simulink model "simulator"  (R2021a)
settings: Solver=ode3  StartTime=0.0  StopTime=5000  FixedStep=1  RelTol=1e-3
InitFcn:
  | clear all
  | clc
  | 
  | %run config_Houston.m
  | run config_Malaga.m
  | 
  | load('PBNsim_buses');
StartFcn:
  | rng('shuffle');
undefined symbols (not defined in the file): entity, initX, instancedAC, m, n, WP, WPabort, WPnext, WPspeed
libraries: AC x23, aerolibactuator x3
(part 2 of 2)

== stateflow chart simulator/ATC/ATC ==
  state COMMUNICATIONS
    entry,during:
    msgProcess
    state msgProcess [function]
      (default) -> (junction 50)
      (junction 50) -> (junction 49) [order 1] : ACmsg
      (junction 48) -> (junction 50)
      (junction 50) -> (junction 53) [order 2]
      (junction 49) -> (junction 48) : {ACmsgProcess}
  data: ATCmsg output Bus: bus_ATMmsg; ACmsg input Bus: bus_ACmsg; WP parameter; WPspeed parameter; WPnext parameter; WPabort parameter
  function ACmsgProcess:
    | function ACmsgProcess
    | coder.extrinsic('delete')
    | coder.extrinsic('get_param')
    | coder.extrinsic('set_param')
    | 
    | persistent emptyAC AC WP2
    | persistent i_plot
    | persistent abortACid abortTime timeFromAbort
    | persistent distfileID logAC
    | 
    | if(isempty(abortACid))
    |   abortACid = 0;
    | end
    | 
    | if(isempty(abortTime))
    |   abortTime = 0;
    | end
    | 
    | if(isempty(timeFromAbort))
    |   timeFromAbort = 0;
    | end
    | 
    | if(isempty(distfileID))
    |     distfileID = fopen('distfile.txt','w');
    | end
    | 
    | if(isempty(logAC))
    |     logAC = fopen('logAC.csv','w');
    | end
    | 
    | 
    | r = 2815;      %radio de giro = 1.52NM en metros
    |  
    | if(isempty(AC))
    | 
    |     emptyAC = struct(                ...
    |        'id',0,                       ...
    |        'x' ,0,'y' ,0,'z' ,0,'psi',0, ...    % posicion y rumbo
    |        'Fs',0,'Vs',0,'Ys',0,         ...    % velocidades
    |        'cWP',0,                      ...    % waypoint actual
    |        'status',1);                         % 1 volando 
    |                                             % 2 en miss app convencional
    |                                             % 3 en miss app con reinyeccion
    |                                             % 4 miss app completado
    |                                             % 5 gap (avión fantasma actuando como hueco)
    |                                             % 6 avion real siguiendo al gemelo Dubins
    |     
    |     % lista de aviones
    |     AC = repmat(emptyAC,50,1); 
    | 
    |     emptyWP = struct(                ...
    |        'pos',[0 0 0],                ...
    |        'speed',0,'next',0);
    |     
    |     % lista de waypoints
    |     WP2 = repmat(emptyWP,50,1); 
    |     
    |     for i = 1:length(WP)
    |         WP2(i).pos   = WP(i,:);
    |         WP2(i).speed = WPspeed(i);
    |         WP2(i).next  = WPnext(i);
    |     end
    |     
    |     % valores de aproximación frustrada
    |     i_plot = 1;
    |     
    | end
    | 
    | % capturo el mensaje
    | ACid      = ACmsg.data.ACid;
    | ACenabled = ACmsg.data.ACenabled;
    | ACx       = ACmsg.data.ACx;
    | ACy       = ACmsg.data.ACy;
    | ACz       = ACmsg.data.ACz;
    | ACpsi     = ACmsg.data.ACpsi;
    | ACaborted = ACmsg.data.ACaborted;
    | discard(ACmsg)
    | 
    | %determino tiempo actual
    | curTime = 0;
    | curTime = get_param('simulator','SimulationTime');
    | 
    | % determino posicion del avion en la lista
    | index = GetACindex(AC,ACid);
    | 
    | % compruebo si el avion esta operativo
    | if ~ACenabled
    |     if index        
    |         if ACid == abortACid
    |             timeFromAbort = curTime - abortTime;
    |             fprintf('%5.0f: aeronave %3.0f aterriza tras abortar el primer intento. Tiempo desde MAPt %4.0f \n', curTime,abortACid, timeFromAbort);
    |             
    |             fclose(distfileID);
    |         end
    |         
    |         AC(index) = emptyAC;   % elimino avion
    |     end
    |     return
    | end
    | 
    | % El avión está en vuelo operativo
    | if ~index
    |     %creamos el avion en la lista
    |     for i = 1:length(AC)
    |         if (AC(i).id == 0)  %hueco libre encontrado
    |             index = i;            
    |             AC(index).id = ACid;     
    |             AC(index).cWP = 2;
    |             break
    |         end
    |     end
    |     if ~index
    |         disp('ERROR: desbordamiento de la tabla de aviones del controlador');
    |         set_param('simulator','SimulationCommand','Stop')
    |     end
    | end
    | 
    | 
    | %Actualiza información del AC
    | if ACid == 5 && ACaborted
    |     % Pintamos la estela del punto
    |     i_plot = i_plot + 1;
    |     if i_plot == 10
    |         i_plot = 1;
    | %         plot3([AC(index).x ACx],...
    | %               [AC(index).y ACy],...
    | %               [AC(index).z ACz],...
    | %               'color',[0.5 0.5 0.5]);
    |         plot3(ACx,ACy,ACz,'.','color',[0.5 0.5 0.5]);
    |     end
    |     
    |     posACaborted = [ACx ACy ACz];
    |     for i = 1:length(AC)
    |         
    |         if (AC(i).id == ACid || AC(i).id==0)
    |             continue
    |         end
    |        
    |         % calcula la distancia entre el avion que aborta y los demas
    |         posACother = [AC(i).x AC(i).y AC(i).z];
    |         Edistance = norm(posACaborted-posACother);
    |         Hdistance = norm([posACaborted(1) posACaborted(2)]-[posACother(1) posACother(2)]);
    |         Vdistance = norm(posACaborted(3)-posACother(3));
    |         fprintf(distfileID,"%4.0f %3.0f %5.0f %5.0f %5.0f\n",...
    |             curTime, AC(i).id,Edistance,Hdistance,Vdistance);
    | %         fprintf('en tiempo %4.0f calculo distancia desde %3.0f a %3.0f: %5.0f m (horizontal: %5.0f m; vertical: %5.0f m)\n',...
    | %             curTime, ACid, AC(i).id,Edistance,Hdistance,Vdistance);
    | %         if (Hdistance < 5556) && (Vdistance < 304.8)
    | %             fprintf('en tiempo %4.0f VIOLACION DE SEPARACIÓN entre %3.0f y %3.0f\n', curTime, ACid, AC(i).id);
    | %         end
    |     end
    | end
    | 
    | 
    | AC(index).x   = ACx;
    | AC(index).y   = ACy;
    | AC(index).z   = ACz;
    | AC(index).psi = ACpsi;
    | 
    | 
    | 
    | %%
    | % compruebo si el avion entra en miss approach
    | if ACaborted && AC(index).status == 1
    |     
    |     % busco hueco disponible
    |     
    |     T1 = 240; % segundos 
    |     T  = 90;  % segundos
    |     w1 = 2;   % waypoint de fin de búsqueda de hueco
    |     g  = GetGap(ACid,T1,T,w1,WP2,AC);
    |     gDir = [sin(g.psi) cos(g.psi)]; 
    |     
    |     if ~g.cWP
    |         
    |         AC(index).status = 2;   % miss app convencional
    | 
    |         abortACid = ACid;
    |         abortTime = get_param('simulator','SimulationTime');
    |         fprintf('%5.0f: aeronave %3.0f ejecuta miss approach convencional\n',abortTime,abortACid);
    | 
    |         AC(index).cWP = WPabort;
    |         ATCmsg.data.ACid    = ACid;
    |         ATCmsg.data.WPx     = WP2(WPabort).pos(1);
    |         ATCmsg.data.WPy     = WP2(WPabort).pos(2);
    |         ATCmsg.data.WPz     = WP2(WPabort).pos(3);
    |         ATCmsg.data.WPspeed = WP2(WPabort).speed;
    |         send(ATCmsg);        
    |         AC(index).status = 4;   % reinjected        
    |         
    |     else
    |         
    |         AC(index).status = 3;   % miss app con reinyección
    |         
    |         %  método de estimación de rumbo:
    |         %  La posición del hueco futura se calcula como el punto de la ruta que:
    |         %  1) el avion reinyectado alcanzaría tras un tiempo t
    |         %  2) el avion trasero alcanzaria tras un tiempo t + (mitad del tiempo con el avion delantero)
    | 
    |         tmin = 0;
    |         tmax = TBA(WP2,AC(index),g);
    |         tcycle = 2*pi*r / (WP2(WPabort).speed * 0.5144); % tiempo empleado en dar una vuelta completa
    |         if tmax < tcycle
    |             disp('ERROR: imposible reinyectar en el hueco proporcionado');
    |             set_param('simulator','SimulationCommand','Stop')
    |         end        
    |         
    |         abortACid = ACid;
    |         abortTime = get_param('simulator','SimulationTime');
    |         fprintf('%5.0f: aeronave %3.0f reinyectada %3.0f segundos detras\n',abortTime,abortACid,tmax);
    |         
    |         threshold  = 1;
    |         tG = 0;  ta = 0;
    |         gePos = [0 0 0]; geDir = [0 0];
    |         WPo = [0 0]; WPd = [0 0]; injWP = 0;
    | %         h_ge = plot3(0,0,0,'o','MarkerFaceColor','none','MarkerEdgeColor','none');
    | 
    |         while tmax-tmin > threshold
    | 
    |             tG = (tmin + tmax) / 2;
    | 
    |             % calculo posición del hueco
    |             [gePos,geDir,injWP] = AdvanceFlight(WP2,g,tG);
    | %             delete(h_ge)
    | %             h_ge = plot3(gePos(1),gePos(2),gePos(3),'o','MarkerFaceColor','none','MarkerEdgeColor','red');
    | 
    |             % calculo tiempo que tarda el avion reinyectado en alcanzar el hueco y el WPi a usar
    |             [ta,WPo,WPd] = Dubins(gePos(1:2),geDir,AC(index),WP2(WPabort).speed,'L');  
    |             ta = max(ta,tcycle);
    |             if (tG < ta)
    |                 tmin = tG; % reducimos el intervalo por abajo
    |             end
    |             if (tG > ta)
    |                 tmax = tG; % reducimos el intervalo por arriba
    |             end
    |         end        
    |    
    |        
    |         c = gePos(1:2) + [-geDir(2) geDir(1)] * r;
    |         ShowTurnRadius(c(1),c(2),r,'green');
    |         
    |         if WPo == [0 0]
    |             disp('ERROR: reinyeccion demasiado proxima');
    |             set_param('simulator','SimulationCommand','Stop')
    |         end 
    | 
    |         % calculo waypoints intermedios
    |         d = norm(gePos(1:2) - WPd);
    |         angle1 = acosd(d / (2*r));
    |         angle3 = (90 - angle1) / 2;
    |         l = tand(angle3)*r;
    | 
    |         Sdir = WPd - WPo;
    |         Sdir = Sdir / norm(Sdir);
    |         WPi1 = WPd + Sdir * l;
    | 
    |         WPi2 = gePos(1:2) - geDir * l;
    | 
    |         
    |         % buscamos hueco para insertar 3 waypoints intermedios
    |         for i = 1:length(WP2)
    |             if WP2(i).speed == 0
    |                 break
    |             end
    |         end
    |         
    |         % creamos waypoint intermedio 1
    |         h_WPi1 = plot3(WPi1(1),WPi1(2),gePos(3),'o','MarkerFaceColor','green','MarkerEdgeColor','none');
    |         WP2(i).pos   = [WPi1 gePos(3)];
    |         WP2(i).speed = WP2(WPabort).speed;
    |         WP2(i).next  = i+1;
    | 
    |         % creamos waypoint intermedio 2
    |         h_WPi2 = plot3(WPi2(1),WPi2(2),gePos(3),'o','MarkerFaceColor','green','MarkerEdgeColor','none');
    |         WP2(i+1).pos   = [WPi2 gePos(3)];
    |         WP2(i+1).speed = WP2(WPabort).speed;
    |         WP2(i+1).next  = i+2;
    | 
    |         % creamos waypoint intermedio 3
    |         h_gePos = plot3(gePos(1),gePos(2),gePos(3),'o','MarkerFaceColor','green','MarkerEdgeColor','none');
    |         WP2(i+2).pos   = gePos;
    |         WP2(i+2).speed = WP2(WPabort).speed;
    |         WP2(i+2).next  = injWP;
    |         
    |         
    |         % salto de waypoint
    |         AC(index).cWP  = i;
    | 
    |         ATCmsg.data.ACid    = ACid;
    |         data = AC(index).cWP;
    |         ATCmsg.data.WPx     = WP2(data).pos(1);
    |         ATCmsg.data.WPy     = WP2(data).pos(2);
    |         ATCmsg.data.WPz     = WP2(data).pos(3);
    |         ATCmsg.data.WPspeed = WP2(data).speed;
    |         send(ATCmsg);         
    |                
    |     end
    |     
    | end
    | 
    | 
    | 
    | %%
    | % Comprobación de si el AC ha alcanzado el waypoint actual
    | 
    | [dist,l] = Distance2WP(WP2,AC(index));
    | speed = WP2(AC(index).cWP).speed * 0.5144; %NM -> m/s
    | if dist < (l + speed*3)
    | 
    |     % Si el avión estaba frustrando, ha alcanzado el waypoint intermedio.
    |     % Por tanto se reinyecta normalmente y debe dejar de calcular hueco.
    |     if AC(index).status == 3
    |         AC(index).status = 4;
    |         
    | %         nWP = WP2(AC(index).cWP).next;
    | %         AC(index).cWP  = nWP;
    |     end
    |     
    |     % salto de waypoint
    | 
    |     nWP = WP2(AC(index).cWP).next;
    |     if nWP
    |         AC(index).cWP  = nWP;
    | 
    |         ATCmsg.data.ACid    = ACid;
    |         ATCmsg.data.WPx     = WP2(nWP).pos(1);
    |         ATCmsg.data.WPy     = WP2(nWP).pos(2);
    |         ATCmsg.data.WPz     = WP2(nWP).pos(3);
    |         ATCmsg.data.WPspeed = WP2(nWP).speed;
    |         send(ATCmsg);
    |     end
    |     
    | end
    | 
    | 
    | % Detección de conflicto de esta aeronave con el resto
    | detectConflict(AC,index);
    | 
    | 
    | 
    | %Inserto registro en log
    | fprintf(logAC,"%05.0f,%03.0f,%1.0f,%+05.2f,%+05.2f,%05.2f,%+1.4f\n" ...
    |              ,curTime           ...
    |              ,ACid              ...
    |              ,AC(index).status  ...
    |              ,ACx,ACy,ACz,ACpsi);
    | 
    | 
    | 
    | end  % function
    | 
    | 
    | %%
    | function index = GetACindex(AC,id)
    |     index = 0;
    |     for i = 1:length(AC)
    |         if (id == AC(i).id)
    |             index = i;            
    |             break
    |         end
    |     end
    | end
    | 
    | %%
    | function index2 = GetNextACindex(AC,index1)
    |     index2 = 0;
    |     nid    = inf;
    |     for i = 1:length(AC)
    |         if (AC(index1).id < AC(i).id) && (AC(i).id < nid)
    |             index2 = i;            
    |             nid    = AC(i).id;
    |         end
    |     end
    | end
    | 
    | %%
    | function g = GetGap(a1index,T1,T,w1,WP2,AC)
    | % Busca un hueco g entre aeronaves
    | %  - para la aeronave a1index
    | %  - con separación T entre ellas
    | %  - tras un tiempo mínimo T1
    | %  - como máximo explora hasta el waypoint w1
    | coder.extrinsic('set_param')
    | 
    | 
    |     % creamos el hueco como una aeronave virtual
    |     g = struct(                ...
    |        'id',0,                       ...
    |        'x' ,0,'y' ,0,'z' ,0,'psi',0, ...    % posicion y rumbo
    |        'Fs',0,'Vs',0,'Ys',0,         ...    % velocidades
    |        'cWP',0,                      ...    % waypoint actual (indica que el hueco no existe)
    |        'status',5);                         % 5 gap (avión fantasma actuando como hueco)
    | 
    |     % Creamos una aeronave virtual en posición del primer waypoint
    |     aWindex  = 0;
    |     for i = 1:length(AC)
    |         if (AC(i).id == 0)  %hueco libre encontrado
    |              aWindex  = i;
    |             break
    |         end
    |     end
    |     if ~aWindex
    |         disp('ERROR: desbordamiento de la tabla de aviones del controlador');
    |         set_param('simulator','SimulationCommand','Stop')
    |     end
    |         
    |     AC(aWindex).id  = 1000000; 
    |     AC(aWindex).x   = WP2(w1).pos(1); 
    |     AC(aWindex).y   = WP2(w1).pos(2); 
    |     AC(aWindex).z   = WP2(w1).pos(3); 
    | 
    |     w2 = WP2(w1).next;
    |     AC(aWindex).cWP = w2;     
    | 
    |     w12 = WP2(w2).pos(1:2) - WP2(w1).pos(1:2);
    |     w12 = w12 / norm(w12);
    |     AC(aWindex).psi = atan2(w12(1),w12(2));
    |     
    |     % buscamos hueco entre aviones
    |     ETA_a1 = ETA(WP2,AC(a1index));
    |     aLindex = a1index;
    |     ETA_aL = ETA_a1;
    | 
    |     while aLindex ~= aWindex
    | 
    |         tL = max(ETA_aL + T, ETA_a1 + T1);
    | 
    |         aFindex = GetNextACindex(AC,aLindex);
    | 
    |         ETA_aF = ETA(WP2,AC(aFindex));
    |         tF = ETA_aF - T;
    |         
    |         if tF > tL - 5     % margen de 5 segundos
    | 
    |             % calculo posición del hueco
    |             gDir = [0 0];
    |             [gapPos,gDir,injWP] = AdvanceFlight(WP2,AC(aFindex),T+tF-tL);
    |             
    |             % asigno hueco
    |             g.x   = gapPos(1);
    |             g.y   = gapPos(2);
    |             g.z   = gapPos(3);
    |             g.psi = atan2(gDir(1),gDir(2));
    |             g.cWP = injWP;
    |             h_gapPos = plot3(g.x,g.y,g.z,'o','MarkerFaceColor','none','MarkerEdgeColor','green');
    | 
    |             break
    |         end
    |         aLindex = aFindex;
    |         ETA_aL  = ETA_aF;
    |     end
    |     
    | end
    | 
    | %%
    | function t = TBA(WP2,ac1,ac2)
    | %Time Between Aircrafts
    | %determina el tiempo existente entre 
    | % (1) el avion delantero 
    | % (2) el avion trasero
    | 
    | %Método
    | % calculamos la diferencia entre los tiempos hasta destino
    |     tac1 = ETA(WP2,ac1);
    |     tac2 = ETA(WP2,ac2);
    |     t = tac2 - tac1;    
    | end
    | 
    | %%
    | function t = ETA(WP2,ac)
    | %Estimated Time to Arrival
    | 
    |     t = 0;
    | 
    |     %obtengo waypoint actual y previo
    |     cWP = ac.cWP;
    |     pWP = 0;
    |     for i = 1:length(WP2)
    |         if (WP2(i).next == cWP)
    |             pWP = i;            
    |             break
    |         end
    |     end
    | 
    |     while ac.cWP ~= 0
    |         % calculo punto de tránsito del WP actual al siguiente
    |         pWPac = struct(               ...
    |             'x'  ,WP2(pWP).pos(1),    ...
    |             'y'  ,WP2(pWP).pos(2),    ...
    |             'cWP',cWP);
    | 
    |         [~,l] = Distance2WP(WP2,pWPac);
    |         
    |         WPdir = WP2(cWP).pos(1:2) - WP2(pWP).pos(1:2);
    |         WPdir = WPdir / norm(WPdir);
    |         ACdir = WPdir;
    |         WPpos = WP2(cWP).pos(1:2) - WPdir*l;
    |         %plot3(WPpos(1),WPpos(2),0,'o','MarkerFaceColor','g','MarkerEdgeColor','none');         
    |         
    |         
    |         [ti,~,~] = Dubins(WPpos,WPdir,ac,WP2(ac.cWP).speed,'LR');
    |         t = t + ti;
    | 
    |         pWP = cWP;
    |         cWP = WP2(cWP).next;
    |         
    |         ac.x   = WPpos(1);
    |         ac.y   = WPpos(2);
    |         ac.psi = atan2(ACdir(1),ACdir(2));
    |         ac.cWP = cWP;        
    | 
    |     end
    |        
    | end
    | 
    | %%
    | function [pos3D,dir2D,fWP] = AdvanceFlight(WP2,ac,t) %version con curvas
    | %Determina donde estará un avión después de un cierto tiempo siguiendo el plan establecido
    | %pos: posición 3D futura del avión
    | %dir: vector 3D unitario en el sentido de avance futuro del avion
    | %fWP: waypoint que seguirá en el futuro
    |   
    | %     if ac.status~=1
    | %         return  % error en la llamada. El avion no va en ruta programada.
    | %     end
    |     
    |     coder.extrinsic('angle2dcm')
    | 
    |     %obtengo waypoint actual y previo
    |     cWP = ac.cWP;
    |     pWP = 0;
    |     for i = 1:length(WP2)
    |         if (WP2(i).next == cWP)
    |             pWP = i;            
    |             break
    |         end
    |     end
    | 
    |     WPo   = [0 0];
    |     WPdir = [0 0];
    |     ACdir = [0 0];
    |     tWP   = 0;
    |     while cWP
    | 
    |         % calculo punto de tránsito del WP actual al siguiente
    |         pWPac = struct(               ...
    |             'x'  ,WP2(pWP).pos(1),    ...
    |             'y'  ,WP2(pWP).pos(2),    ...
    |             'cWP',cWP);
    | 
    |         [~,l] = Distance2WP(WP2,pWPac);
    |         
    |         WPdir = WP2(cWP).pos(1:2) - WP2(pWP).pos(1:2);
    |         WPdir = WPdir / norm(WPdir);
    |         ACdir = WPdir;
    |         WPpos = WP2(cWP).pos(1:2) - WPdir*l;
    |         %plot3(WPpos(1), WPpos(2),WPpos(3),'o','MarkerFaceColor','g','MarkerEdgeColor','none');    
    | 
    |         % Determino la curva de Dubins óptima
    |         [tWP,WPo,~]  = Dubins(WPpos,WPdir,ac,WP2(cWP).speed,'LR');
    | 
    |         if tWP < t
    |             pWP = cWP;
    |             cWP = WP2(cWP).next;
    |             t   = t - tWP;
    | 
    |             ac.x   = WPpos(1);
    |             ac.y   = WPpos(2);
    |             ac.psi = atan2(ACdir(1),ACdir(2));
    |             ac.cWP = cWP;
    |         else
    |             break
    |         end
    |     end
    |         
    |     % Ya no llegaremos al siguiente waypoint
    |     
    |     % calculo la altura futura
    |     pWPh = WP2(pWP).pos(3);
    |     cWPh = WP2(cWP).pos(3);
    |     descenso = (pWPh - cWPh)* t/tWP;
    |     h = pWPh - descenso;
    |      
    |     % calculo la posición horizontal
    |     [tWPo,~,~] = Dubins(WPo,WPdir,ac,WP2(cWP).speed,'LR');
    |     if t < tWPo %la posición futura está en el tramo curvo
    | 
    | %         axis([-39164   -29995    35162    44330])
    | %         plot3(ac.x, ac.y,0,'+')
    | %         plot3(WPo(1), WPo(2),0,'+')
    |         
    |         % calculo ángulo a rotar
    |         angleAC2WP = acos(dot(ACdir,WPdir));
    |         angle = angleAC2WP * t/tWPo;
    |         
    |         %calculo vector radio
    |         r  = 2815; %radio de giro = 1.52NM en metros
    |         cAC = [sin(ac.psi+pi/2) cos(ac.psi+pi/2)] * r; 
    | 
    |         izqder = cross([ACdir 0],[WPdir 0]);
    |         if izqder(3) < 0
    |             %giro a derecha
    |             cAC   = -cAC; 
    |             angle = -angle;
    |         end
    |         
    |         %calculo centro de circunferencia de rotación
    |         c  =  [ac.x ac.y] - cAC;
    | %         h1 = ShowTurnRadius(c(1),c(2),r,'green');
    |         
    |         %roto vectores el angulo indicado
    |         mr = angle2dcm(angle,0,0);
    | 
    |         cACrot = [0 0 0];
    |         cACrot = [cAC 0] * mr;
    |         pos2D = cACrot(1:2) + c;
    |         
    |         ACdirrot = [ACdir 0] * mr;
    |         dir2D = ACdirrot(1:2);
    |         
    |     else %la posición futura está en el tramo recto
    | 
    |         t = t - tWPo;
    |         speed = WP2(cWP).speed * 0.5144; %NM -> m/s
    |         pos2D = WPo + WPdir * speed * t;
    |         dir2D = WPdir;
    |         
    |     end
    |     
    |     pos3D = [pos2D h];
    |     fWP = ac.cWP;
    |     
    | end
    | 
    | %%
    | function [t,WPo,WPd] = Dubins(Tpos,Tdir,ac,speed, mode)
    | %Determina el tiempo que tardaría un avión para alcanzar una posición determinada
    | %mediante un giro, una recta, y un giro
    | %t: tiempo que tardaría
    | %WPo: waypoint 2D: fin    de maniobra de giro inicial
    | %WPd: waypoint 2D: inicio de maniobra de giro final
    | %Tpos: posición 2D objetivo
    | %Tdir: dirección 2D objetivo
    | %ac: datos del avión
    | %speed: velocidad en nudos a utilizar
    | %mode: indico si la maniobra debe ser a izquierda, derecha, o da igual
    |     
    |     t = inf;
    |     WPo = [0 0];
    |     WPd = [0 0];
    |     
    |     % determino si están tan cerca que no es posible hacer Dubins
    |     dist = norm(Tpos - [ac.x ac.y]);
    |     r = 2815; %radio de giro = 1.52NM en metros
    |     if dist < r
    |         t = dist / (speed * 0.5144);  %nudos -> m/s
    |         return
    |     end
    | 
    |     % Determino la curva de Dubins óptima
    |     if contains(mode,'L')
    |         [t, WPo, WPd ] = Dubins_LSL(Tpos,Tdir,ac,speed);
    |         [t2,WPo2,WPd2] = Dubins_LSR(Tpos,Tdir,ac,speed);  
    |         if (t2 < t)
    |             t   = t2;
    |             WPo = WPo2;
    |             WPd = WPd2;
    |         end
    |     end
    | 
    |     if contains(mode,'R')
    |         [t2,WPo2,WPd2] = Dubins_RSL(Tpos,Tdir,ac,speed);  
    |         if (t2 < t)
    |             t   = t2;
    |             WPo = WPo2;
    |             WPd = WPd2;
    |         end
    |         [t2,WPo2,WPd2] = Dubins_RSR(Tpos,Tdir,ac,speed);
    |         if (t2 < t)
    |             t   = t2;
    |             WPo = WPo2;
    |             WPd = WPd2;
    |         end 
    |     end
    | end
    | 
    | %%
    | function [t,WPo,WPd] = Dubins_LSL(Tpos,Tdir,ac,speed)
    | %Determina el tiempo que tardaría un avión para alcanzar una posición determinada
    | %mediante un giro a izquierda, una recta, y un giro a la izquierda
    | %t: tiempo que tardaría
    | %WPo: waypoint 2D: fin    de maniobra de giro inicial
    | %WPd: waypoint 2D: inicio de maniobra de giro final
    | %Tpos: posición 2D objetivo
    | %Tdir: dirección 2D objetivo
    | %ac: datos del avión
    | %speed: velocidad en nudos a utilizar
    | 
    |     r = 2815; %radio de giro = 1.52NM en metros
    | 
    |     % circunferencia de origen
    |     coAC = [sin(ac.psi+pi/2) cos(ac.psi+pi/2)]; 
    |     co   =  [ac.x ac.y] - coAC * r;
    |     h1   = ShowTurnRadius(co(1),co(2),r,'green');
    |     
    |     % circunferencia de destino
    |     cdT  = [Tdir(2) -Tdir(1)] / norm(Tdir); 
    |     cd   = Tpos - cdT * r;
    |     h2   = ShowTurnRadius(cd(1),cd(2),r,'blue');
    | 
    |     % cocd: vector unitario de circunferencia origen a circunferencia destino
    |     cocd = cd - co;
    |     s2   = norm(cocd);       % longitud del segmento en línea recta
    |     if s2 > 1
    |         %caso normal:
    |         %circunferencias de origen y destino distintas
    |         
    |         cocd = cocd/s2;
    | 
    |         % waypoint intermedio de origen
    |         cS  = [cocd(2) -cocd(1)];
    |         WPo = co + cS * r;
    |         h3  = plot3(WPo(1), WPo(2),0,'o','MarkerFaceColor','g','MarkerEdgeColor','none');    
    | 
    |         % waypoint intermedio de destino
    |         WPd = cd + cS * r;
    |         h4  = plot3(WPd(1), WPd(2),0,'o','MarkerFaceColor','g','MarkerEdgeColor','none');    
    |         h5  = plot3([WPd(1) WPo(1)],[WPd(2) WPo(2)],[0 0],'b','Color','red');
    | 
    |         % longitud del segmento curvo de origen
    |         ao = AngleTurningRight(cS,coAC);
    |         if rad2deg(ao) > 330
    |             %Evitamos dar una vuelta en círculo
    |             ao = ao - 2*pi;
    |             WPo = [ac.x ac.y];
    |         end
    |         s1 = ao * r;
    | 
    |         % longitud del segmento curvo de destino
    |         ad = AngleTurningRight(cdT,cS);
    |         if rad2deg(ad) > 330
    |             %Evitamos dar una vuelta en círculo
    |             ad = ad - 2*pi;
    |             WPd = Tpos;
    |         end
    |         s3 = ad * r;
    |         
    |     else
    |         %caso particular:
    |         %circunferencias de origen y destino coincidentes
    | 
    |         % waypoint intermedio de origen
    |         WPo = [ac.x ac.y];
    |         h3  = plot3(WPo(1), WPo(2),0,'o','MarkerFaceColor','g','MarkerEdgeColor','none');    
    | 
    |         % waypoint intermedio de destino
    |         WPd = [ac.x ac.y];
    |         h4  = plot3(WPd(1), WPd(2),0,'o','MarkerFaceColor','g','MarkerEdgeColor','none');    
    |         h5  = plot3([WPd(1) WPo(1)],[WPd(2) WPo(2)],[0 0],'b','Color','red');
    | 
    |         % longitud del segmento curvo de origen
    |         s1 = 0;
    | 
    |         % longitud del segmento curvo de destino
    |         ad = AngleTurningRight(cdT,coAC);
    |         s3 = ad * r;
    | 
    |     end
    |     
    |     %velocidad
    |     speed = speed * 0.5144;           %nudos -> m/s
    |     
    |     %tiempo
    |     t = (s1+s2+s3)/speed;
    |     
    |     coder.extrinsic('delete')
    |     delete([h1 h2 h3 h4 h5])
    | 
    | end
    | 
    | %%
    | function [t,WPo,WPd] = Dubins_RSL(Tpos,Tdir,ac,speed)
    | %Determina el tiempo que tardaría un avión para alcanzar una posición determinada
    | %mediante un giro a derecha, una recta, y un giro a la izquierda
    | %t: tiempo que tardaría
    | %WPo: waypoint 2D: fin    de maniobra de giro inicial
    | %WPd: waypoint 2D: inicio de maniobra de giro final
    | %Tpos: posición 2D objetivo
    | %Tdir: dirección 2D objetivo
    | %ac: datos del avión
    | %speed: velocidad en nudos a utilizar
    | 
    |     coder.extrinsic('delete')
    | 
    |     r = 2815; %radio de giro = 1.52NM en metros
    | 
    |     % circunferencia de origen
    |     coAC = [sin(ac.psi-pi/2) cos(ac.psi-pi/2)]; 
    |     co   = [ac.x ac.y] - coAC * r;
    |     h1   = ShowTurnRadius(co(1),co(2),r,'green');
    |     
    |     % circunferencia de destino
    |     cdT  = [Tdir(2) -Tdir(1)] / norm(Tdir); 
    |     cd   = Tpos - cdT * r;
    |     h2   = ShowTurnRadius(cd(1),cd(2),r,'blue');
    | 
    | 
    |     % cocd: vector unitario de circunferencia origen a circunferencia destino
    |     cocd = cd - co;
    |     d  = norm(cocd);
    |     cocd = cocd/d;
    |     if (d < 2*r) 
    |         %las circunferencias intersecan
    |         %por tanto no hay solución con tangentes internas
    |         t = inf;
    |         WPo = [0 0];
    |         WPd = [0 0];
    |         delete([h1 h2])
    |         return
    |     end
    |     
    |     % waypoint intermedio de origen
    |     cocdn = [-cocd(2) cocd(1)];
    |     alpha = acos(2*r/d);
    |     coS   = cocd*cos(alpha) + cocdn*sin(alpha);
    |     WPo   = co + coS * r;
    |     h3    = plot3(WPo(1), WPo(2),0,'o','MarkerFaceColor','g','MarkerEdgeColor','none');    
    | 
    |     % waypoint intermedio de destino
    |     cdS = -coS;
    |     WPd = cd + cdS * r;
    |     h4  = plot3(WPd(1), WPd(2),0,'o','MarkerFaceColor','g','MarkerEdgeColor','none');    
    |     h5  = plot3([WPd(1) WPo(1)],[WPd(2) WPo(2)],[0 0],'b','Color','red');
    |     
    |     % longitud del segmento curvo de origen
    |     ao = AngleTurningRight(coAC,coS);
    |     if rad2deg(ao) > 330
    |         %Evitamos dar una vuelta en círculo
    |         ao = ao - 2*pi;
    |         WPo = [ac.x ac.y];
    |     end
    |     s1 = ao * r;
    |     
    |     % longitud del segmento en línea recta
    |     s2 = sqrt(d^2 - (2*r)^2);
    |      
    |     % longitud del segmento curvo de destino
    |     ad = AngleTurningRight(cdT,cdS);
    |     if rad2deg(ad) > 330
    |         %Evitamos dar una vuelta en círculo
    |         ad = ad - 2*pi;
    |         WPd = Tpos;
    |     end
    |     s3 = ad * r;
    |     
    |     %velocidad
    |     speed = speed * 0.5144;           %nudos -> m/s
    |     
    |     %tiempo
    |     t = (s1+s2+s3)/speed;
    |     
    |     delete([h1 h2 h3 h4 h5])
    | 
    | end
    | 
    | %%
    | function [t,WPo,WPd] = Dubins_RSR(Tpos,Tdir,ac,speed)
    | %Determina el tiempo que tardaría un avión para alcanzar una posición determinada
    | %mediante un giro a derecha, una recta, y un giro a la derecha
    | %t: tiempo que tardaría
    | %WPo: waypoint 2D: fin    de maniobra de giro inicial
    | %WPd: waypoint 2D: inicio de maniobra de giro final
    | %Tpos: posición 2D objetivo
    | %Tdir: dirección 2D objetivo
    | %ac: datos del avión
    | %speed: velocidad en nudos a utilizar
    | 
    |     coder.extrinsic('delete')
    | 
    |     r = 2815; %radio de giro = 1.52NM en metros
    | 
    |     % circunferencia de origen
    |     coAC = [sin(ac.psi-pi/2) cos(ac.psi-pi/2)]; 
    |     co   =  [ac.x ac.y] - coAC * r;
    |     h1   = ShowTurnRadius(co(1),co(2),r,'green');
    |     
    |     % circunferencia de destino
    |     cdT  = [-Tdir(2) Tdir(1)] / norm(Tdir); 
    |     cd   = Tpos - cdT * r;
    |     h2   = ShowTurnRadius(cd(1),cd(2),r,'blue');
    | 
    |     % cocd: vector unitario de circunferencia origen a circunferencia destino
    |     cocd = cd - co;
    |     s2   = norm(cocd);       % longitud del segmento en línea recta
    |     
    |     if s2 > 1
    |         %caso normal:
    |         %circunferencias de origen y destino distintas
    | 
    |         cocd = cocd/s2;
    | 
    |         % waypoint intermedio de origen
    |         cS  = [-cocd(2) cocd(1)];
    |         WPo = co + cS * r;
    |         h3  = plot3(WPo(1), WPo(2),0,'o','MarkerFaceColor','green','MarkerEdgeColor','none');    
    | 
    |         % waypoint intermedio de destino
    |         WPd = cd + cS * r;
    |         h4  = plot3(WPd(1), WPd(2),0,'o','MarkerFaceColor','blue','MarkerEdgeColor','none');    
    |         h5  = plot3([WPd(1) WPo(1)],[WPd(2) WPo(2)],[0 0],'b','Color','red');
    | %         h6 = plot3([cd(1) cd(1)+cS(1)*r],[cd(2) cd(2)+cS(2)*r],[0 0],'b','Color','blue');
    | %         h7 = plot3([cd(1) cd(1)+cdT(1)*r],[cd(2) cd(2)+cdT(2)*r],[0 0],'b','Color','red');    
    | 
    |         % longitud del segmento curvo de origen
    |         thetao = AngleTurningRight(coAC,cS);
    |         if rad2deg(thetao) > 330
    |             %Evitamos dar una vuelta en círculo
    |             thetao = thetao - 2*pi;
    |             WPo = [ac.x ac.y];
    |         end
    |         s1 = thetao * r;
    | 
    |         % longitud del segmento curvo de destino
    |         thetad = AngleTurningRight(cS,cdT);
    |         if rad2deg(thetad) > 330
    |             %Evitamos dar una vuelta en círculo
    |             thetad = thetad - 2*pi;
    |             WPd = Tpos;
    |         end
    |         s3 = thetad * r;
    |         
    |     else
    |         %caso particular:
    |         %circunferencias de origen y destino coincidentes
    | 
    |         % waypoint intermedio de origen
    |         WPo = [ac.x ac.y];
    |         h3  = plot3(WPo(1), WPo(2),0,'o','MarkerFaceColor','g','MarkerEdgeColor','none');    
    | 
    |         % waypoint intermedio de destino
    |         WPd = [ac.x ac.y];
    |         h4  = plot3(WPd(1), WPd(2),0,'o','MarkerFaceColor','g','MarkerEdgeColor','none');    
    |         h5  = plot3([WPd(1) WPo(1)],[WPd(2) WPo(2)],[0 0],'b','Color','red');
    |         
    |         % longitud del segmento curvo de origen
    |         s1 = 0;
    | 
    |         % longitud del segmento curvo de destino
    |         thetad = AngleTurningRight(coAC,cdT);
    |         s3 = thetad * r;
    |         
    |     end
    |     
    |     
    |     %velocidad
    |     speed = speed * 0.5144;           %nudos -> m/s
    |     
    |     %tiempo
    |     t = (s1+s2+s3)/speed;
    |     
    |     delete([h1 h2 h3 h4 h5])
    | 
    | end
    | 
    | %%
    | function [t,WPo,WPd] = Dubins_LSR(Tpos,Tdir,ac,speed)
    | %Determina el tiempo que tardaría un avión para alcanzar una posición determinada
    | %mediante un giro a izquierda, una recta, y un giro a la derecha
    | %t: tiempo que tardaría
    | %WPo: waypoint 2D: fin    de maniobra de giro inicial
    | %WPd: waypoint 2D: inicio de maniobra de giro final
    | %Tpos: posición 2D objetivo
    | %Tdir: dirección 2D objetivo
    | %ac: datos del avión
    | %speed: velocidad en nudos a utilizar
    | 
    |     coder.extrinsic('delete')
    | 
    |     r = 2815; %radio de giro = 1.52NM en metros
    | 
    |     % circunferencia de origen
    |     coAC = [sin(ac.psi+pi/2) cos(ac.psi+pi/2)]; 
    |     co   = [ac.x ac.y] - coAC * r;
    |     h1   = ShowTurnRadius(co(1),co(2),r,'green');
    |     
    |     % circunferencia de destino
    |     cdT  = [-Tdir(2) Tdir(1)] / norm(Tdir); 
    |     cd   = Tpos - cdT * r;
    |     h2   = ShowTurnRadius(cd(1),cd(2),r,'blue');
    | 
    | 
    |     % cocd: vector unitario de circunferencia origen a circunferencia destino
    |     cocd = cd - co;
    |     d  = norm(cocd);
    |     cocd = cocd/d;
    |     if (d < 2*r) 
    |         %las circunferencias intersecan
    |         %por tanto no hay solución con tangentes internas
    |         t = inf;
    |         WPo = [0 0];
    |         WPd = [0 0];
    |         delete([h1 h2])
    |         return
    |     end
    |     
    |     % waypoint intermedio de origen
    |     cocdn = [cocd(2) -cocd(1)];
    |     alpha = acos(2*r/d);
    |     coS   = cocd*cos(alpha) + cocdn*sin(alpha);
    |     WPo   = co + coS * r;
    |     h3    = plot3(WPo(1), WPo(2),0,'o','MarkerFaceColor','g','MarkerEdgeColor','none');    
    | 
    |     % waypoint intermedio de destino
    |     cdS = -coS;
    |     WPd = cd + cdS * r;
    |     h4  = plot3(WPd(1), WPd(2),0,'o','MarkerFaceColor','g','MarkerEdgeColor','none');    
    |     h5  = plot3([WPd(1) WPo(1)],[WPd(2) WPo(2)],[0 0],'b','Color','red');
    |     
    |     % longitud del segmento curvo de origen
    |     ao = AngleTurningRight(coS,coAC);
    |     if rad2deg(ao) > 330
    |         %Evitamos dar una vuelta en círculo
    |         ao = ao - 2*pi;
    |         WPo = [ac.x ac.y];
    |     end
    |     s1 = ao * r;
    |     
    |     % longitud del segmento en línea recta
    |     s2 = sqrt(d^2 - (2*r)^2);
    |      
    |     % longitud del segmento curvo de destino
    |     ad = AngleTurningRight(cdS,cdT);
    |     if rad2deg(ad) > 330
    |         %Evitamos dar una vuelta en círculo
    |         ad = ad - 2*pi;
    |         WPd = Tpos;
    |     end
    |     s3 = ad * r;
    |     
    |     %velocidad
    |     speed = speed * 0.5144;           %nudos -> m/s
    |     
    |     %tiempo
    |     t = (s1+s2+s3)/speed;
    |     
    |     delete([h1 h2 h3 h4 h5])
    | 
    | end
    | 
    | %%
    | function [dist,l] = Distance2WP(WP2,ac)
    | % dist: distancia al waypoint (se asume que volamos directamente hacia él)
    | % l: distancia a la que habría que virar rumbo al siguiente waypoint
    | 
    |     r = 2815; %radio de giro = 1.52NM en metros
    | 
    |     % calculo distancia hasta el WP actual
    |     cWP = ac.cWP;
    |     vec_AC_cWP = WP2(cWP).pos(1:2)-[ac.x ac.y];
    |     dist = norm(vec_AC_cWP);
    | 
    |     % Si existen más waypoint tras el actual... calculo distancia a la que virar
    |     nWP = WP2(ac.cWP).next;
    |     if nWP~=0
    |         %calculo vector currentWP -> nextWP
    |         vec_cWP_nWP = WP2(nWP).pos(1:2) - WP2(cWP).pos(1:2);
    |         %calculo angulo entre segmentos
    |         num = dot(-vec_AC_cWP,vec_cWP_nWP);
    |         den = dist*norm(vec_cWP_nWP);
    |         theta = acos(num/den);  % colocados con el mismo origen
    |         alpha = pi - theta;     % colocados consecutivamente
    |         l = r * tan(alpha/2);   % distancia al WP para empezar el giro
    |     else
    |         l = 0;
    |     end
    |     
    | end
    | 
    | %%
    | function handle = ShowTurnRadius(xc,yc,r,color)
    |         %pinto circulo de radio r
    |         t=0:pi/30:2*pi;
    |         x=cos(t)*r + xc;
    |         y=sin(t)*r + yc;
    |         handle = plot(x,y,'Color',color);
    | end
    |         
    | %%
    | function a12 = AngleTurningRight (v1,v2)
    | % ángulo resultante de girar v1 hacia la derecha hasta encontrar a v2
    | 
    |     a1 = atan2d(v1(1),v1(2));
    |     a1 = mod(a1,360);
    | 
    |     a2 = atan2d(v2(1),v2(2));
    |     a2 = mod(a2,360);
    |     
    |     if(a2 < a1)
    |         a2 = a2 + 360;
    |     end
    |     a12 = a2-a1;
    |     a12 = deg2rad(a12);
    | end
    | 
    | %%
    | 
    | function [indexC,Vdist,Hdist,time] = detectConflict(AC,index)
    |     coder.extrinsic('get_param');
    | 
    |     indexC = 0;
    |     ac1 = AC(index);
    |     for i = 1:length(AC)
    |         if (i == index) || (AC(i).id == 0)
    |             continue
    |         end
    |         Vdist = ac1.z - AC(i).z;
    |         Hdist = norm([ac1.x ac1.y] - [AC(i).x AC(i).y]);
    |         if (Vdist < 304.8) && (Hdist < 5556)
    |             indexC = i;
    |             time = get_param('simulator','SimulationTime');
    |             break
    |         end
    |     end
    |     
    |     if indexC == 0
    |         Vdist = 0;
    |         Hdist = 0;
    |         time  = 0;
    |     end        
    |     
    | end

== stateflow chart simulator/Air Space/AC05/pilot ==
  state NAVIGATOR [parallel]
    settings: executionOrder=1
    state WAKEUP
      entry:
      wakeUp
    state OFF
      entry:
      reset
    state SLEEP
      entry:
      sleep
    state FLY
      entry, during:
      follow
    (default) -> OFF
    OFF -> WAKEUP : [flightInfo.ACenabled]
    SLEEP -> OFF
    WAKEUP -> FLY
    FLY -> SLEEP : [landed]
  state COMUNICATIONS [parallel]
    updateRadar
    settings: executionOrder=2
  data: resp function_output; imuDubins input; cmdDubins input; imu input; cmd output Bus: bus_command; flightInfo input Bus: bus_ADSB; radar output Bus: bus_radar; ACid local double; cWP local; dist local; WP parameter; WPspeed parameter; ACenabled local; ACaborted local
  function wakeUp:
    | function wakeUp
    | 
    | % inicializo navegación
    | ACid = flightInfo.ACid;
    | ACenabled = 1;
    | cWP = [WP(2,:) WPspeed(2)];
  function reset:
    | function reset
    | 
    | % reseteo estado de la aeronave
    | ACid = 0;
    | ACenabled = 0;
    | ACaborted = 0;
    | 
    | % reseteo movimiento
    | coder.extrinsic('convvel');
    | cmd.Fa = 123.4667; %convvel(cWP(4),'kts','m/s'); %123 m/s
    | cmd.Vs = 0;
    | cmd.Ys = 0;
  function sleep:
    | function sleep
    | 
    | % Desactivamos el avión y dejamos que pase un ciclo 
    | % ara que el RADAR lo elimine
    | ACenabled = 0;
  function follow:
    | function follow
    | 
    | p = [imuDubins.ACx-imu.ACx, imuDubins.ACy-imu.ACy];
    | 
    | alpha = imuDubins.ACpsi + cmdDubins.Ys;
    | F = [sin(alpha) cos(alpha)] * cmdDubins.Fa;
    | 
    | Fp = (F*60 + p) / 60;
    | cmd.Fa = norm(Fp);
    | alphap = atan2(Fp(1),Fp(2));
    |     
    | cmd.Ys = AngleBetweenOrientations(imu.ACpsi,alphap);
    | cmd.Ys = min(cmd.Ys,+0.05);
    | cmd.Ys = max(cmd.Ys,-0.05);
    | 
    | dz   = imuDubins.ACz - imu.ACz;    
    | kV  = 0.1;
    | varVs = kV * dz;
    | cmd.Vs = cmdDubins.Vs + varVs;
    | 
    | end
    | 
    | function a12 = AngleBetweenOrientations (or1,or2)
    | % ángulo mas corto desde la orientación or1 a la orientación or2
    | 
    |     or1 = rad2deg(or1);
    |     or1 = mod(or1,360);
    |  
    |     or2 = rad2deg(or2);
    |     or2 = mod(or2,360);
    | 
    |     a12 = or2-or1;
    | 
    |     if(a12 > 180)
    |         a12 = a12 - 360;
    |     end
    |     if(a12 < -180)
    |         a12 = a12 + 360;
    |     end
    | 
    |     a12 = deg2rad(a12);
    | end
  function resp = landed:
    | function resp = landed
    | % Concluye si el avion ha terminado de recorrer la pista
    | 
    | resp = false;
    | 
    | if imu.ACz < 50 % estamos a menos de 50 metros de altura
    |     %busco WP con velocidad 50 (solo el último la tiene)
    |     fWP = WP(find(WPspeed==50,1),:);
    |     %calculo segmento desde el AC a este WP
    |     s = fWP(1:2)-[imu.ACx imu.ACy];
    |     dist = norm(s);
    |     if dist < 50
    |         resp = true;
    |     end
    | end
  function updateRadar:
    | function updateRadar
    | 
    | radar.ACid      = ACid;
    | radar.ACenabled = ACenabled;
    | radar.ACdubins  = 0;
    | 
    | radar.ACx       = imu.ACx;
    | radar.ACy       = imu.ACy;
    | radar.ACz       = imu.ACz;
    | radar.ACpsi     = imu.ACpsi;
    | 
    | 
    | 
    | 
    | 
    | %% Grabo movimiento en el fichero de LOG
    | 
    | persistent logAC
    | if(isempty(logAC))
    |     logAC = fopen('logAC.csv','w');
    | end
    | 
    | coder.extrinsic('get_param')
    | curTime = get_param('simulator','SimulationTime');
    | 
    | %Inserto registro en log
    | fprintf(logAC,"%05.0f,%03.0f,%1.0f,%+05.2f,%+05.2f,%05.2f,%+1.4f\n" ...
    |              ,curTime           ...
    |              ,ACid              ...
    |              ,6                 ...  % AC(index).status = 6 (real AC)
    |              ,imu.ACx           ...
    |              ,imu.ACy           ...
    |              ,imu.ACz           ...
    |              ,imu.ACpsi);
